simulink model "filter_FIR"  (R2020a)
settings: Solver=VariableStepAuto  StartTime=0.0  StopTime=10.0  RelTol=1e-3
libraries: simulink x1
settings Model: Creator=INDRAJIT MARATHE  LastModifiedBy=INDRAJIT MARATHE

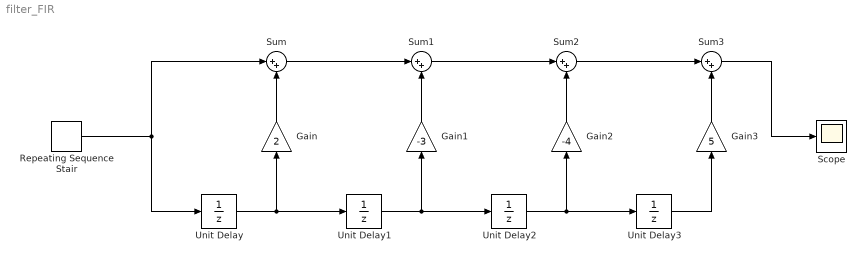
== system filter_FIR ==
  Gain : Gain  Gain=2
  Gain1 : Gain  Gain=-3
  Gain2 : Gain  Gain=-4
  Gain3 : Gain  Gain=5
  Repeating Sequence Stair : simulink/Sources/Repeating Sequence Stair  OutValues=[3 1 4 2 1].'  tsamp=-1  OutMin=[]  OutMax=[]  OutDataTypeStr=double  OutputDataTypeScalingMode=double  OutDataType=fixdt(0,8)  ConRadixGroup=Best Precision: Vector-wise  OutScaling=2^-12
  Scope : Scope
  Sum{,1..3} (4 alike) : Sum  Inputs=|++
  Unit Delay{,1..3} (4 alike) : UnitDelay  SampleTime=-1  HasFrameUpgradeWarning=on
  wires:
  Gain/1 -> Sum/2
  Repeating Sequence Stair/1 -> Sum/1, Unit Delay/1
  Sum/1 -> Sum1/1
  Gain1/1 -> Sum1/2
  Unit Delay/1 -> Gain/1, Unit Delay1/1
  Sum1/1 -> Sum2/1
  Gain2/1 -> Sum2/2
  Unit Delay1/1 -> Unit Delay2/1, Gain1/1
  Sum2/1 -> Sum3/1
  Unit Delay3/1 -> Gain3/1
  Gain3/1 -> Sum3/2
  Unit Delay2/1 -> Gain2/1, Unit Delay3/1
  Sum3/1 -> Scope/1
